simulink library "csc_psr_process_slant_range_lib"  (R2015b)
settings: Solver=VariableStepAuto  StartTime=0.0  StopTime=10.0  RelTol=1e-3
undefined symbols (not defined in the file or in its folder): central_body_flattening, central_body_radius, central_body_rotation_rate, ini_topocentric_latitude, kfl_target_site_planet_fixed, lander_dcm
undefined symbols (not defined in the file): lander_pos
libraries: util_common_lib x12, simulink_extras x6, util_frame_rotation_lib x6, simulink x4, util_fsw_frame_rotation_lib x4, util_quat_lib x4, util_geodesy_lib x4
settings Model: Creator=Mark Agbayani  LastModifiedBy=Mark Agbayani

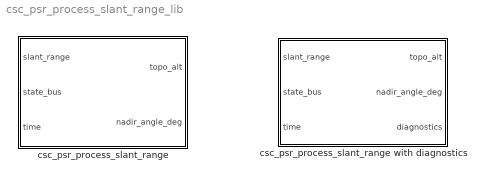
== system csc_psr_process_slant_range_lib ==
  csc_psr_process_slant_range : Subsystem  mask{position_in_lander=lander_pos, lander_dcm=lander_dcm}
      mask prompts: position_in_lander "LIDAR Position in Body Frame (meters)"; lander_dcm "LIDAR Attitude wrt Body Frame (DCM)"
  csc_psr_process_slant_range with diagnostics : Subsystem  mask{position_in_lander=lander_pos, lander_dcm=lander_dcm}
      mask prompts: position_in_lander "LIDAR Position in Body Frame (meters)"; lander_dcm "LIDAR Attitude wrt Body Frame (DCM)"

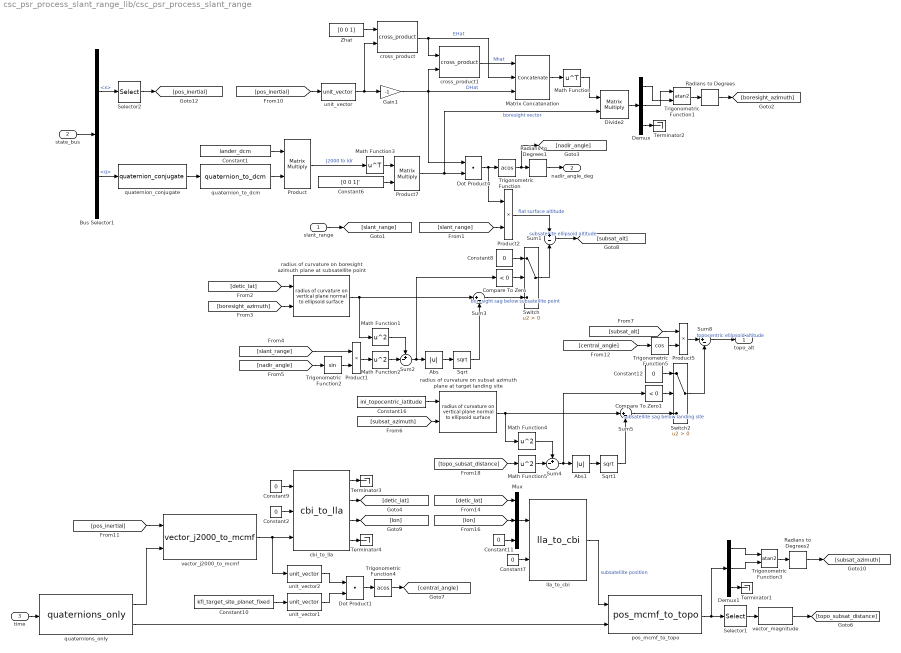
== system csc_psr_process_slant_range_lib/csc_psr_process_slant_range ==
  slant_range : Inport
  state_bus : Inport  Port=2
  time : Inport  Port=3
  Abs : Abs
  Abs1 : Abs
  Bus Selector1 : BusSelector  OutputSignals=x,q
  Compare To Zero : simulink/Logic and Bit Operations/Compare To Zero  relop=<  OutDataTypeStr=boolean
  Compare To Zero1 : simulink/Logic and Bit Operations/Compare To Zero  relop=<  OutDataTypeStr=boolean
  Constant1 : Constant  Value=lander_dcm
  Constant10 : Constant  Value=kfl_target_site_planet_fixed
  Constant{2,7..9,11..12} (6 alike) : Constant  Value=0
  Constant16 : Constant  Value=ini_topocentric_latitude
  Constant6 : Constant  Value=[0 0 1]'  VectorParams1D=off
  Demux : Demux  Outputs=3
  Demux1 : Demux  Outputs=3
  Divide2 : Product  Inputs=**  Multiplication=Matrix(*)
  Dot Product1 : DotProduct  InputSameDT=on  OutDataTypeStr=Inherit: Inherit via internal rule
  Dot Product4 : DotProduct  InputSameDT=on  OutDataTypeStr=Inherit: Inherit via internal rule
  Gain1 : Gain  Gain=-1
  Math Function : Math  Operator=transpose  SaturateOnIntegerOverflow=on
  Math Function{1..2,4..5} (4 alike) : Math  Operator=square  SaturateOnIntegerOverflow=on
  Math Function3 : Math  Operator=transpose  SaturateOnIntegerOverflow=on
  Matrix Concatenation : Concatenate  NumInputs=3  Mode=Multidimensional array  ConcatenateDimension=2
  Mux : Mux  Inputs=3
  Product : Product  Multiplication=Matrix(*)  RndMeth=Zero
  Product1 : Product  Inputs=**  RndMeth=Zero
  Product2 : Product  Inputs=**  RndMeth=Zero
  Product5 : Product  Inputs=**  RndMeth=Zero
  Product7 : Product  Multiplication=Matrix(*)  RndMeth=Zero
  Radians to Degrees : simulink_extras/Transformations/Radians to Degrees
  Radians to Degrees1 : simulink_extras/Transformations/Radians to Degrees
  Radians to Degrees2 : simulink_extras/Transformations/Radians to Degrees
  Selector1 : Selector  InputPortWidth=3  IndexOptions=Index vector (dialog)  Indices=[1 2]  OutputSizes=1
  Selector2 : Selector  InputPortWidth=kfl_n_state  IndexOptions=Index vector (dialog)  Indices=kfl_pos_index  OutputSizes=1
  Sqrt : Sqrt  SaturateOnIntegerOverflow=on
  Sqrt1 : Sqrt  SaturateOnIntegerOverflow=on
  Sum1 : Sum  Inputs=+|-
  Sum2 : Sum  Inputs=+-|  AccumDataTypeStr=double
  Sum3 : Sum  Inputs=|+-
  Sum4 : Sum  Inputs=+-|  AccumDataTypeStr=double
  Sum5 : Sum  Inputs=|+-
  Sum8 : Sum  Inputs=|+-
  Switch : Switch  Criteria=u2 > Threshold
  Switch2 : Switch  Criteria=u2 > Threshold
  Terminator{1..4} (4 alike) : Terminator
  Trigonometric Function : Trigonometry  Operator=acos
  Trigonometric Function1 : Trigonometry  Operator=atan2
  Trigonometric Function2 : Trigonometry
  Trigonometric Function3 : Trigonometry  Operator=atan2
  Trigonometric Function4 : Trigonometry  Operator=acos
  Trigonometric Function5 : Trigonometry  Operator=cos
  Zhat : Constant  Value=[0 0 1]
  cbi_to_lla : util_frame_rotation_lib/cbi_to_lla  a=central_body_radius  b=central_body_radius*(1-central_body_flattening)  omega=central_body_rotation_rate(3)
  cross_product : util_common_lib/cross_product  SystemSampleTime=-1
  cross_product1 : util_common_lib/cross_product  SystemSampleTime=-1
  lla_to_cbi : util_frame_rotation_lib/lla_to_cbi  a=central_body_radius  b=central_body_radius*(1-central_body_flattening)
  pos_mcmf_to_topo : util_fsw_frame_rotation_lib/pos_mcmf_to_topo  SystemSampleTime=-1
  quaternion_conjugate : util_quat_lib/quaternion_conjugate  SystemSampleTime=-1
  quaternion_to_dcm : util_quat_lib/quaternion_to_dcm  SystemSampleTime=-1
  quaternions_only : util_frame_rotation_lib/quaternions_only  SystemSampleTime=-1
  radius of curvature on boresight azimuth plane at subsatellite point : util_geodesy_lib/radius of curvature on vertical plane normal to ellipsoid surface  a=central_body_radius  b=central_body_radius*(1-central_body_flattening)
  radius of curvature on subsat azimuth plane at target landing site : util_geodesy_lib/radius of curvature on vertical plane normal to ellipsoid surface  a=central_body_radius  b=central_body_radius*(1-central_body_flattening)
  unit_vector : util_common_lib/unit_vector  SystemSampleTime=-1
  unit_vector1 : util_common_lib/unit_vector  SystemSampleTime=-1
  unit_vector2 : util_common_lib/unit_vector  SystemSampleTime=-1
  vector_j2000_to_mcmf : util_fsw_frame_rotation_lib/vector_j2000_to_mcmf  SystemSampleTime=-1
  vector_magnitude : util_common_lib/vector_magnitude  SystemSampleTime=-1
  topo_alt : Outport
  nadir_angle_deg : Outport  Port=2
  wires:
  Bus Selector1/1 -> Selector2/1  "<x>"
  Bus Selector1/2 -> quaternion_conjugate/1  "<q>"
  Product/1 -> Math Function3/1  "J2000 to ldr"
  Math Function3/1 -> Product7/1
  quaternion_to_dcm/1 -> Product/2
  Constant1/1 -> Product/1
  Constant6/1 -> Product7/2
  quaternion_conjugate/1 -> quaternion_to_dcm/1
  Dot Product4/1 -> Product2/1, Trigonometric Function/1
  Trigonometric Function/1 -> [nadir_angle], Radians to Degrees1/1
  Radians to Degrees1/1 -> nadir_angle_deg/1
  Product7/1 -> Dot Product4/2, Divide2/2  "boresight vector"
  state_bus/1 -> Bus Selector1/1
  Demux/2 -> Trigonometric Function1/1
  Demux/1 -> Trigonometric Function1/2
  Trigonometric Function1/1 -> Radians to Degrees/1
  Divide2/1 -> Demux/1
  Math Function/1 -> Divide2/1
  Zhat/1 -> cross_product/1
  Matrix Concatenation/1 -> Math Function/1
  cross_product1/1 -> Matrix Concatenation/1  "Nhat"
  cross_product/1 -> cross_product1/1, Matrix Concatenation/2  "EHat"
  Gain1/1 -> Matrix Concatenation/3, Dot Product4/1, cross_product1/2  "DHat"
  Radians to Degrees/1 -> [boresight_azimuth]
  unit_vector/1 -> Gain1/1, cross_product/2
  Demux/3 -> Terminator2/1
  Sum8/1 -> topo_alt/1  "topocentric ellipsoid altitude"
  radius of curvature on subsat azimuth plane at target landing site/1 -> Math Function4/1, Sum5/1
  Math Function4/1 -> Sum4/1
  Math Function5/1 -> Sum4/2
  Sqrt1/1 -> Sum5/2
  Sum5/1 -> Switch2/3  "subsatellite sag below landing site"
  Compare To Zero1/1 -> Switch2/2
  Constant12/1 -> Switch2/1
  Abs1/1 -> Sqrt1/1
  Sum4/1 -> Compare To Zero1/1, Abs1/1
  [topo_subsat_distance] -> Math Function5/1
  Trigonometric Function5/1 -> Product5/2
  [subsat_alt] -> Product5/1
  [central_angle] -> Trigonometric Function5/1
  Product5/1 -> Sum8/1
  Switch2/1 -> Sum8/2
  Constant16/1 -> radius of curvature on subsat azimuth plane at target landing site/1
  [subsat_azimuth] -> radius of curvature on subsat azimuth plane at target landing site/2
  Product2/1 -> Sum1/1  "flat surface altitude"
  [detic_lat] -> radius of curvature on boresight azimuth plane at subsatellite point/1
  [boresight_azimuth] -> radius of curvature on boresight azimuth plane at subsatellite point/2
  radius of curvature on boresight azimuth plane at subsatellite point/1 -> Sum3/1, Math Function1/1
  Math Function1/1 -> Sum2/1
  Math Function2/1 -> Sum2/2
  Sqrt/1 -> Sum3/2
  [nadir_angle] -> Trigonometric Function2/1
  Trigonometric Function2/1 -> Product1/2
  Product1/1 -> Math Function2/1
  [slant_range] -> Product1/1
  Sum1/1 -> [subsat_alt]  "subsatellite ellipsoid altitude"
  Sum3/1 -> Switch/3  "boresight sag below subsatellite point"
  Compare To Zero/1 -> Switch/2
  Constant8/1 -> Switch/1
  Abs/1 -> Sqrt/1
  Sum2/1 -> Abs/1, Compare To Zero/1
  Switch/1 -> Sum1/2
  time/1 -> quaternions_only/1
  Dot Product1/1 -> Trigonometric Function4/1
  Constant10/1 -> unit_vector1/1
  Trigonometric Function4/1 -> [central_angle]
  Selector1/1 -> vector_magnitude/1
  quaternions_only/1 -> vector_j2000_to_mcmf/2
  quaternions_only/2 -> pos_mcmf_to_topo/2
  lla_to_cbi/1 -> pos_mcmf_to_topo/1  "subsatellite position"
  vector_magnitude/1 -> [topo_subsat_distance]
  Mux/1 -> lla_to_cbi/1
  cbi_to_lla/4 -> Terminator4/1
  Constant7/1 -> lla_to_cbi/2
  Trigonometric Function3/1 -> Radians to Degrees2/1
  Demux1/3 -> Terminator1/1
  pos_mcmf_to_topo/1 -> Demux1/1, Selector1/1
  Radians to Degrees2/1 -> [subsat_azimuth]
  Demux1/1 -> Trigonometric Function3/1
  Demux1/2 -> Trigonometric Function3/2
  vector_j2000_to_mcmf/1 -> unit_vector2/1, cbi_to_lla/3
  Constant2/1 -> cbi_to_lla/2
  Constant9/1 -> cbi_to_lla/1
  cbi_to_lla/1 -> Terminator3/1
  cbi_to_lla/3 -> [lon]
  cbi_to_lla/2 -> [detic_lat]
  [lon] -> Mux/2
  [detic_lat] -> Mux/1
  Constant11/1 -> Mux/3
  unit_vector1/1 -> Dot Product1/2
  [pos_inertial] -> vector_j2000_to_mcmf/1
  unit_vector2/1 -> Dot Product1/1
  Selector2/1 -> [pos_inertial]
  [pos_inertial] -> unit_vector/1
  [slant_range] -> Product2/2
  slant_range/1 -> [slant_range]

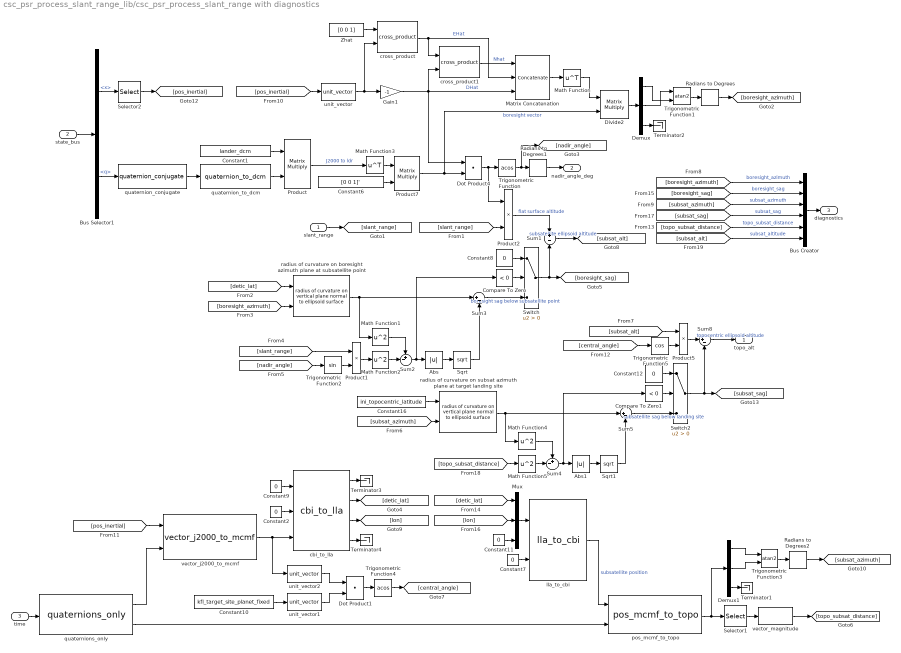
== system csc_psr_process_slant_range_lib/csc_psr_process_slant_range with diagnostics ==
  slant_range : Inport
  state_bus : Inport  Port=2
  time : Inport  Port=3
  Abs : Abs
  Abs1 : Abs
  Bus Creator : BusCreator  Inputs=6
  Bus Selector1 : BusSelector  OutputSignals=x,q
  Compare To Zero : simulink/Logic and Bit Operations/Compare To Zero  relop=<  OutDataTypeStr=boolean
  Compare To Zero1 : simulink/Logic and Bit Operations/Compare To Zero  relop=<  OutDataTypeStr=boolean
  Constant1 : Constant  Value=lander_dcm
  Constant10 : Constant  Value=kfl_target_site_planet_fixed
  Constant{2,7..9,11..12} (6 alike) : Constant  Value=0
  Constant16 : Constant  Value=ini_topocentric_latitude
  Constant6 : Constant  Value=[0 0 1]'  VectorParams1D=off
  Demux : Demux  Outputs=3
  Demux1 : Demux  Outputs=3
  Divide2 : Product  Inputs=**  Multiplication=Matrix(*)
  Dot Product1 : DotProduct  InputSameDT=on  OutDataTypeStr=Inherit: Inherit via internal rule
  Dot Product4 : DotProduct  InputSameDT=on  OutDataTypeStr=Inherit: Inherit via internal rule
  Gain1 : Gain  Gain=-1
  Math Function : Math  Operator=transpose  SaturateOnIntegerOverflow=on
  Math Function{1..2,4..5} (4 alike) : Math  Operator=square  SaturateOnIntegerOverflow=on
  Math Function3 : Math  Operator=transpose  SaturateOnIntegerOverflow=on
  Matrix Concatenation : Concatenate  NumInputs=3  Mode=Multidimensional array  ConcatenateDimension=2
  Mux : Mux  Inputs=3
  Product : Product  Multiplication=Matrix(*)  RndMeth=Zero
  Product1 : Product  Inputs=**  RndMeth=Zero
  Product2 : Product  Inputs=**  RndMeth=Zero
  Product5 : Product  Inputs=**  RndMeth=Zero
  Product7 : Product  Multiplication=Matrix(*)  RndMeth=Zero
  Radians to Degrees : simulink_extras/Transformations/Radians to Degrees
  Radians to Degrees1 : simulink_extras/Transformations/Radians to Degrees
  Radians to Degrees2 : simulink_extras/Transformations/Radians to Degrees
  Selector1 : Selector  InputPortWidth=3  IndexOptions=Index vector (dialog)  Indices=[1 2]  OutputSizes=1
  Selector2 : Selector  InputPortWidth=kfl_n_state  IndexOptions=Index vector (dialog)  Indices=kfl_pos_index  OutputSizes=1
  Sqrt : Sqrt  SaturateOnIntegerOverflow=on
  Sqrt1 : Sqrt  SaturateOnIntegerOverflow=on
  Sum1 : Sum  Inputs=+|-
  Sum2 : Sum  Inputs=+-|  AccumDataTypeStr=double
  Sum3 : Sum  Inputs=|+-
  Sum4 : Sum  Inputs=+-|  AccumDataTypeStr=double
  Sum5 : Sum  Inputs=|+-
  Sum8 : Sum  Inputs=|+-
  Switch : Switch  Criteria=u2 > Threshold
  Switch2 : Switch  Criteria=u2 > Threshold
  Terminator{1..4} (4 alike) : Terminator
  Trigonometric Function : Trigonometry  Operator=acos
  Trigonometric Function1 : Trigonometry  Operator=atan2
  Trigonometric Function2 : Trigonometry
  Trigonometric Function3 : Trigonometry  Operator=atan2
  Trigonometric Function4 : Trigonometry  Operator=acos
  Trigonometric Function5 : Trigonometry  Operator=cos
  Zhat : Constant  Value=[0 0 1]
  cbi_to_lla : util_frame_rotation_lib/cbi_to_lla  a=central_body_radius  b=central_body_radius*(1-central_body_flattening)  omega=central_body_rotation_rate(3)
  cross_product : util_common_lib/cross_product  SystemSampleTime=-1
  cross_product1 : util_common_lib/cross_product  SystemSampleTime=-1
  lla_to_cbi : util_frame_rotation_lib/lla_to_cbi  a=central_body_radius  b=central_body_radius*(1-central_body_flattening)
  pos_mcmf_to_topo : util_fsw_frame_rotation_lib/pos_mcmf_to_topo  SystemSampleTime=-1
  quaternion_conjugate : util_quat_lib/quaternion_conjugate  SystemSampleTime=-1
  quaternion_to_dcm : util_quat_lib/quaternion_to_dcm  SystemSampleTime=-1
  quaternions_only : util_frame_rotation_lib/quaternions_only  SystemSampleTime=-1
  radius of curvature on boresight azimuth plane at subsatellite point : util_geodesy_lib/radius of curvature on vertical plane normal to ellipsoid surface  a=central_body_radius  b=central_body_radius*(1-central_body_flattening)
  radius of curvature on subsat azimuth plane at target landing site : util_geodesy_lib/radius of curvature on vertical plane normal to ellipsoid surface  a=central_body_radius  b=central_body_radius*(1-central_body_flattening)
  unit_vector : util_common_lib/unit_vector  SystemSampleTime=-1
  unit_vector1 : util_common_lib/unit_vector  SystemSampleTime=-1
  unit_vector2 : util_common_lib/unit_vector  SystemSampleTime=-1
  vector_j2000_to_mcmf : util_fsw_frame_rotation_lib/vector_j2000_to_mcmf  SystemSampleTime=-1
  vector_magnitude : util_common_lib/vector_magnitude  SystemSampleTime=-1
  topo_alt : Outport
  nadir_angle_deg : Outport  Port=2
  diagnostics : Outport  Port=3
  wires:
  [subsat_alt] -> Bus Creator/6  "subsat_altitude"
  Bus Selector1/1 -> Selector2/1  "<x>"
  Bus Selector1/2 -> quaternion_conjugate/1  "<q>"
  Product/1 -> Math Function3/1  "J2000 to ldr"
  Math Function3/1 -> Product7/1
  quaternion_to_dcm/1 -> Product/2
  Constant1/1 -> Product/1
  Constant6/1 -> Product7/2
  quaternion_conjugate/1 -> quaternion_to_dcm/1
  Dot Product4/1 -> Product2/1, Trigonometric Function/1
  Trigonometric Function/1 -> [nadir_angle], Radians to Degrees1/1
  Radians to Degrees1/1 -> nadir_angle_deg/1
  Product7/1 -> Dot Product4/2, Divide2/2  "boresight vector"
  state_bus/1 -> Bus Selector1/1
  Demux/2 -> Trigonometric Function1/1
  Demux/1 -> Trigonometric Function1/2
  Trigonometric Function1/1 -> Radians to Degrees/1
  Divide2/1 -> Demux/1
  Math Function/1 -> Divide2/1
  Zhat/1 -> cross_product/1
  Matrix Concatenation/1 -> Math Function/1
  cross_product1/1 -> Matrix Concatenation/1  "Nhat"
  cross_product/1 -> cross_product1/1, Matrix Concatenation/2  "EHat"
  Gain1/1 -> Matrix Concatenation/3, Dot Product4/1, cross_product1/2  "DHat"
  Radians to Degrees/1 -> [boresight_azimuth]
  unit_vector/1 -> Gain1/1, cross_product/2
  Demux/3 -> Terminator2/1
  Sum8/1 -> topo_alt/1  "topocentric ellipsoid altitude"
  radius of curvature on subsat azimuth plane at target landing site/1 -> Math Function4/1, Sum5/1
  Math Function4/1 -> Sum4/1
  Math Function5/1 -> Sum4/2
  Sqrt1/1 -> Sum5/2
  Sum5/1 -> Switch2/3  "subsatellite sag below landing site"
  Compare To Zero1/1 -> Switch2/2
  Constant12/1 -> Switch2/1
  Abs1/1 -> Sqrt1/1
  Sum4/1 -> Compare To Zero1/1, Abs1/1
  [topo_subsat_distance] -> Math Function5/1
  Trigonometric Function5/1 -> Product5/2
  [subsat_alt] -> Product5/1
  [central_angle] -> Trigonometric Function5/1
  Product5/1 -> Sum8/1
  Switch2/1 -> [subsat_sag], Sum8/2
  Constant16/1 -> radius of curvature on subsat azimuth plane at target landing site/1
  [subsat_azimuth] -> radius of curvature on subsat azimuth plane at target landing site/2
  Product2/1 -> Sum1/1  "flat surface altitude"
  [detic_lat] -> radius of curvature on boresight azimuth plane at subsatellite point/1
  [boresight_azimuth] -> radius of curvature on boresight azimuth plane at subsatellite point/2
  radius of curvature on boresight azimuth plane at subsatellite point/1 -> Sum3/1, Math Function1/1
  Math Function1/1 -> Sum2/1
  Math Function2/1 -> Sum2/2
  Sqrt/1 -> Sum3/2
  [nadir_angle] -> Trigonometric Function2/1
  Trigonometric Function2/1 -> Product1/2
  Product1/1 -> Math Function2/1
  [slant_range] -> Product1/1
  Sum1/1 -> [subsat_alt]  "subsatellite ellipsoid altitude"
  Sum3/1 -> Switch/3  "boresight sag below subsatellite point"
  Compare To Zero/1 -> Switch/2
  Constant8/1 -> Switch/1
  Abs/1 -> Sqrt/1
  Sum2/1 -> Abs/1, Compare To Zero/1
  Switch/1 -> [boresight_sag], Sum1/2
  time/1 -> quaternions_only/1
  Dot Product1/1 -> Trigonometric Function4/1
  Constant10/1 -> unit_vector1/1
  Trigonometric Function4/1 -> [central_angle]
  Selector1/1 -> vector_magnitude/1
  quaternions_only/1 -> vector_j2000_to_mcmf/2
  quaternions_only/2 -> pos_mcmf_to_topo/2
  lla_to_cbi/1 -> pos_mcmf_to_topo/1  "subsatellite position"
  vector_magnitude/1 -> [topo_subsat_distance]
  Mux/1 -> lla_to_cbi/1
  cbi_to_lla/4 -> Terminator4/1
  Constant7/1 -> lla_to_cbi/2
  Trigonometric Function3/1 -> Radians to Degrees2/1
  Demux1/3 -> Terminator1/1
  pos_mcmf_to_topo/1 -> Demux1/1, Selector1/1
  Radians to Degrees2/1 -> [subsat_azimuth]
  Demux1/1 -> Trigonometric Function3/1
  Demux1/2 -> Trigonometric Function3/2
  vector_j2000_to_mcmf/1 -> unit_vector2/1, cbi_to_lla/3
  Constant2/1 -> cbi_to_lla/2
  Constant9/1 -> cbi_to_lla/1
  cbi_to_lla/1 -> Terminator3/1
  cbi_to_lla/3 -> [lon]
  cbi_to_lla/2 -> [detic_lat]
  [lon] -> Mux/2
  [detic_lat] -> Mux/1
  Constant11/1 -> Mux/3
  unit_vector1/1 -> Dot Product1/2
  [pos_inertial] -> vector_j2000_to_mcmf/1
  unit_vector2/1 -> Dot Product1/1
  Selector2/1 -> [pos_inertial]
  [pos_inertial] -> unit_vector/1
  [slant_range] -> Product2/2
  slant_range/1 -> [slant_range]
  Bus Creator/1 -> diagnostics/1
  [boresight_azimuth] -> Bus Creator/1  "boresight_azimuth"
  [boresight_sag] -> Bus Creator/2  "boresight_sag"
  [topo_subsat_distance] -> Bus Creator/5  "topo_subsat_distance"
  [subsat_azimuth] -> Bus Creator/3  "subsat_azimuth"
  [subsat_sag] -> Bus Creator/4  "subsat_sag"
